simulink model "Level2"  (R2012b)
settings: Solver=FixedStepDiscrete  StartTime=0.0  StopTime=50  RelTol=1e-3
InitFcn:
  | N=256;
  | Fs = 1000;
  | bw = 5.6;
undefined symbols (not defined in the file): gcbh, rmidispblock
settings Model: RequirementInfo={'other' '..\..\..\requirements\ebd_srs.doc' '@Simulink_requirement_level2' 'true' '3.1.3.3 Level 2 PD' '' } %GIDa_c6020189_f7f2_4521_8d61_041236f87344  Creator=aanantha  LastModifiedBy=klindqvi
settings DataIOCC: SaveFormat=Structure  SignalLoggingSaveFormat=ModelDataLogs  SaveOutput=off  SaveTime=off  SignalLoggingName=logsOut
settings OptimizationCC: InlineParams=on  OptimizeModelRefInitCode=on  LifeSpan=1
settings DebuggingCC: ReadBeforeWriteMsg=DisableAll  WriteAfterWriteMsg=DisableAll  WriteAfterReadMsg=DisableAll  SolverPrmCheckMsg=none  InheritedTsInSrcMsg=none  ParameterPrecisionLossMsg=none  FcnCallInpInsideContextMsg=EnableAllAsWarning
settings HardwareCC: ProdLargestAtomicInteger=Long  ProdLargestAtomicFloat=Double  ProdEndianess=LittleEndian  ProdHWDeviceType=ARM Compatible->ARM Cortex
settings RTWCC: SystemTargetFile=ert.tlc  TemplateMakefile=ert_default_tmf  Description=Embedded Coder  GenerateReport=on  RTWVerbose=off  ProcessScript=ert_make_rtw_hook  IncludeHyperlinkInReport=on  LaunchReport=on  PortableWordSizes=on  CodeProfilingSaveOptions=AllData  GenerateTraceInfo=on  GenerateTraceReportSl=on  GenerateTraceReportSf=on  GenerateTraceReportEml=on  GenerateCodeMetricsReport=on
settings CodeAppCC: IgnoreCustomStorageClasses=off
settings ERTTargetCC: CodeReplacementLibrary=GCC ARM Cortex-A8  MultiwordLength=2048  GenerateSampleERTMain=on  ERTCustomFileTemplate=example_file_process.tlc  ConvertIfToSwitch=off  SuppressUnreachableDefaultCases=off

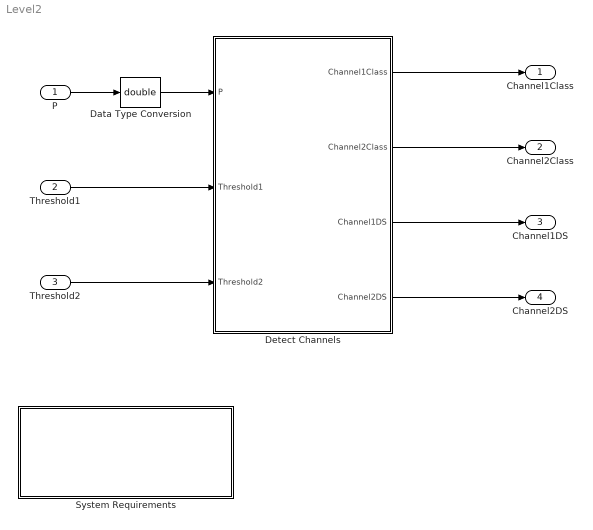
== system Level2 ==
  P : Inport  OutDataTypeStr=single  PortDimensions=1  SampleTime=[0.08900000000000001,0]
  Threshold1 : Inport  Port=2  OutDataTypeStr=double  PortDimensions=1  SampleTime=[0.08900000000000001,0]
  Threshold2 : Inport  Port=3  OutDataTypeStr=double  PortDimensions=1  SampleTime=[0.08900000000000001,0]
  Data Type Conversion : DataTypeConversion  OutDataTypeStr=double
  Detect Channels : Subsystem  RequirementInfo={} %GIDa_bf0bf25c_22e1_4e45_9ba5_31703b9cd88e
  System Requirements : Subsystem  LoadFcn=rmidispblock('load',gcbh)  mask(System Requirements){id=SystemReq, title=System Requirements}
      mask prompts: title "Block Title"
      mask help: Lists the requirements for the current model.
      mask init:
      | id = 'SystemReq';
      | [w,h] = rmidispblock('display',gcbh);
      settings: CopyFcn=rmidispblock('create',gcbh)  DeleteFcn=rmidispblock('delete',gcbh)  ModelCloseFcn=rmidispblock('close',gcbh)  PreSaveFcn=rmidispblock('close',gcbh)  PostSaveFcn=rmidispblock('open',gcbh)  OpenFcn=rmidispblock('open',gcbh)  MoveFcn=rmidispblock('move',gcbh)
      mask Help: helpview(fullfile(docroot,'toolbox','slvnv','slvnv.map'),'systemrequirements')
      mask Display: text(w/2,h-4,rmidispblock('title',gcbh),'horizontalAlignment','center','verticalAlignment','top')
  Channel1Class : Outport  OutDataTypeStr=boolean  PortDimensions=1  SampleTime=[0.08900000000000001,0]
  Channel2Class : Outport  Port=2  OutDataTypeStr=boolean  PortDimensions=1  SampleTime=[0.08900000000000001,0]
  Channel1DS : Outport  Port=3  OutDataTypeStr=double  PortDimensions=1  SampleTime=[0.08900000000000001,0]
  Channel2DS : Outport  Port=4  OutDataTypeStr=double  PortDimensions=1  SampleTime=[0.08900000000000001,0]
  wires:
  P/1 -> Data Type Conversion/1
  Threshold1/1 -> Detect Channels/2(Threshold1)
  Threshold2/1 -> Detect Channels/3(Threshold2)
  Detect Channels/1(Channel1Class) -> Channel1Class/1
  Detect Channels/2(Channel2Class) -> Channel2Class/1
  Detect Channels/3(Channel1DS) -> Channel1DS/1
  Detect Channels/4(Channel2DS) -> Channel2DS/1
  Data Type Conversion/1 -> Detect Channels/1(P)

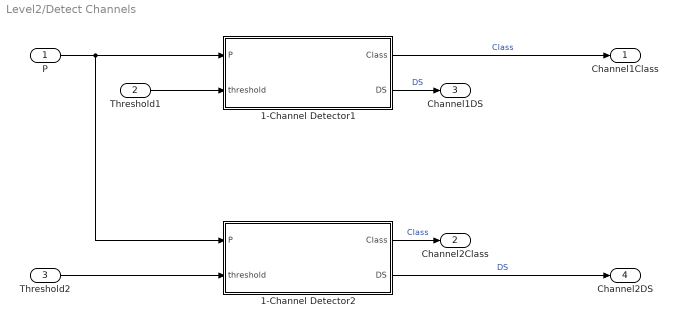
== system Level2/Detect Channels ==
  P : Inport
  Threshold1 : Inport  Port=2
  Threshold2 : Inport  Port=3
  1-Channel Detector1 : MATLAB Function  TreatAsAtomicUnit=on
  1-Channel Detector2 : MATLAB Function  TreatAsAtomicUnit=on
  Channel1Class : Outport
  Channel2Class : Outport  Port=2
  Channel1DS : Outport  Port=3
  Channel2DS : Outport  Port=4
  wires:
  1-Channel Detector2/2(DS) -> Channel2DS/1  "DS"
  Threshold2/1 -> 1-Channel Detector2/2(threshold)
  Threshold1/1 -> 1-Channel Detector1/2(threshold)
  P/1 -> 1-Channel Detector1/1(P), 1-Channel Detector2/1(P)
  1-Channel Detector1/1(Class) -> Channel1Class/1  "Class"
  1-Channel Detector1/2(DS) -> Channel1DS/1  "DS"
  1-Channel Detector2/1(Class) -> Channel2Class/1  "Class"

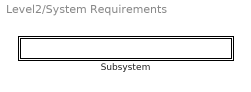
== system Level2/System Requirements ==
  Subsystem : Subsystem  mask{label=0, index=1}
      mask init:
      | label = rmidispblock('label',index);
      settings: OpenFcn=rmidispblock('openReq',gcbh);
      mask Display: text(0,0,label,'horizontalAlignment','left','verticalAlignment','bottom')

== system Level2/System Requirements/Subsystem ==

== matlab function Level2/Detect Channels/1-Channel Detector2 ==
  data: P input; Class output boolean; DS output; threshold input
function [Class,DS] = channelDetector(P, threshold) %#codegen

% Maintain running Noise and Signal History
persistent Noise Signal  sCount nCount

% Gains for initializing the Signal/Noise History
initSignalLevelGain = 1.1;
initNoiseLevelGain = 0.9;

% Counters to maintain running average of histories
sCount = 1; 
nCount = 1;

if isempty(Noise)
    % Noise Level
    Noise = P * initNoiseLevelGain;
    nCount = 1; 
end

if isempty(Signal)
    % Signal Level
    Signal = P * initSignalLevelGain;
    sCount = 1; 
end

DS = (P-Noise)/(Signal-Noise); 

% Limit Value of Detection Strength to between 0 and 1
if DS > 1
    DS(1) = 1;
elseif DS <0
    DS(1) = 0; 
end

% Update Signal/Noise Histories
if DS > threshold
    % Classify as Signal and update Signal History
    Class = true; %boolean(1);  % a-Beat
    Signal = (Signal*sCount + P) / (sCount+1);
    sCount = sCount + 1; 
else
    % Classify as Noise and update Noise History
    Class = false; % not-a-Beat
    Signal = (Signal*nCount + P) / (nCount+1);   
    nCount = nCount + 1; 
end

== matlab function Level2/Detect Channels/1-Channel Detector1 ==
  data: P input; Class output boolean; DS output; threshold input
function [Class,DS] = channelDetector(P, threshold) %#codegen

% Maintain running Noise and Signal History
persistent Noise Signal sCount nCount

% Gains for initializing the Signal/Noise History
initSignalLevelGain = 1.1;
initNoiseLevelGain = 0.9;

% Counters to maintain running average of histories


if isempty(Noise)
    % Noise Level
    Noise = P * initNoiseLevelGain;
    nCount = 1;
end

if isempty(Signal)
    % Signal Level
    Signal = P * initSignalLevelGain;
    sCount = 1; 
end

DS = (P-Noise)/(Signal-Noise); 

% Limit Value of Detection Strength to between 0 and 1
if DS > 1
    DS = 1;
elseif DS <0
    DS = 0; 
end

% Update Signal/Noise Histories
if DS > threshold
    % Classify as Signal and update Signal History
    Class = true; %boolean(1);  % a-Beat
    Signal = (Signal*sCount + P) / (sCount+1);
    sCount = sCount + 1; 
else
    % Classify as Noise and update Noise History
    Class = false; % not-a-Beat
    Signal = (Signal*nCount + P) / (nCount+1);   
    nCount = nCount + 1; 
end
